simulink model "model"  (R2023a)
settings: Solver=VariableStepAuto  StartTime=0.0  StopTime=10.0  RelTol=1e-3
settings Model: Creator=Theomur  LastModifiedBy=пользователь

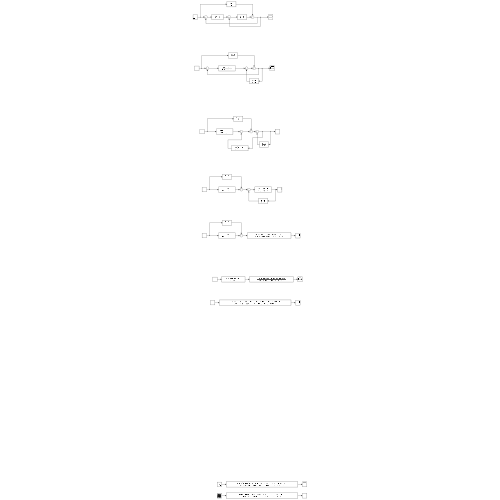
[thumbnail: Simulink's stored preview of the top-level diagram]
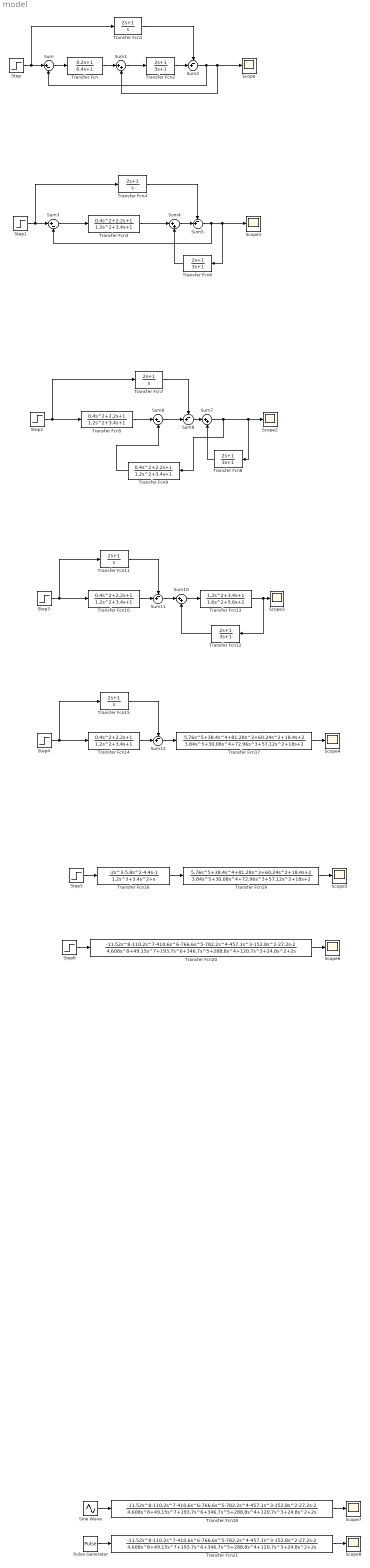
== system model ==
  Pulse Generator : DiscretePulseGenerator  PulseType=Time based  Period=10  PulseWidth=5
  Scope{,1..8} (9 alike) : Scope
  Sine Wave : Sin  SampleTime=0
  Step{,1..6} (7 alike) : Step  SampleTime=0
  Sum : Sum  Inputs=|+-
  Sum{1,4,7,10} (4 alike) : Sum  Inputs=|++
  Sum{2,5,8,11..12} (5 alike) : Sum  Inputs=-+|
  Sum3 : Sum  Inputs=|+-
  Sum6 : Sum  Inputs=|+-
  Transfer Fcn : TransferFcn  Numerator=[0.2 1]  Denominator=[0.4 1]
  Transfer Fcn{1,4,7,11,15} (5 alike) : TransferFcn  Numerator=[2 1]  Denominator=[1 0]
  Transfer Fcn{3,5,9..10,14} (5 alike) : TransferFcn  Numerator=[0.4 2.2 1]  Denominator=[1.2 3.4 1]
  Transfer Fcn{2,6,8,12} (4 alike) : TransferFcn  Numerator=[2 1]  Denominator=[3 1]
  Transfer Fcn13 : TransferFcn  Numerator=[1.2 3.4 1]  Denominator=[1.6 5.6 2]
  Transfer Fcn16 : TransferFcn  Numerator=[-2 -5.8 -4.4 -1]  Denominator=[1.2 3.4 1 0]
  Transfer Fcn17 : TransferFcn  Numerator=[5.76 38.4 81.28 60.24 18.4 2]  Denominator=[3.84 30.08 72.96 57.12 18 2]
  Transfer Fcn18 : TransferFcn  Numerator=[-11.52 -110.2 -410.6 -766.6 -782.2 -457.1 -152.8 -27.2 -2]  Denominator=[4.608 49.15 193.7 346.7 288.8 120.7 24.8 2 0]
  Transfer Fcn19 : TransferFcn  Numerator=[5.76 38.4 81.28 60.24 18.4 2]  Denominator=[3.84 30.08 72.96 57.12 18 2]
  Transfer Fcn20 : TransferFcn  Numerator=[-11.52 -110.2 -410.6 -766.6 -782.2 -457.1 -152.8 -27.2 -2]  Denominator=[4.608 49.15 193.7 346.7 288.8 120.7 24.8 2 0]
  Transfer Fcn21 : TransferFcn  Numerator=[-11.52 -110.2 -410.6 -766.6 -782.2 -457.1 -152.8 -27.2 -2]  Denominator=[4.608 49.15 193.7 346.7 288.8 120.7 24.8 2 0]
  wires:
  Step/1 -> Transfer Fcn1/1, Sum/1
  Sum/1 -> Transfer Fcn/1
  Transfer Fcn/1 -> Sum1/1
  Sum1/1 -> Transfer Fcn2/1
  Sum2/1 -> Sum/2, Scope/1, Sum1/2
  Transfer Fcn2/1 -> Sum2/2
  Transfer Fcn1/1 -> Sum2/1
  Transfer Fcn4/1 -> Sum5/1
  Sum5/1 -> Sum3/2, Transfer Fcn6/1, Scope1/1
  Step1/1 -> Transfer Fcn4/1, Sum3/1
  Sum3/1 -> Transfer Fcn3/1
  Sum4/1 -> Sum5/2
  Transfer Fcn3/1 -> Sum4/1
  Transfer Fcn6/1 -> Sum4/2
  Transfer Fcn8/1 -> Sum7/2
  Step2/1 -> Transfer Fcn7/1, Transfer Fcn5/1
  Sum7/1 -> Transfer Fcn9/1, Transfer Fcn8/1, Scope2/1
  Transfer Fcn7/1 -> Sum8/1
  Sum8/1 -> Sum7/1
  Transfer Fcn5/1 -> Sum6/1
  Sum6/1 -> Sum8/2
  Transfer Fcn9/1 -> Sum6/2
  Step3/1 -> Transfer Fcn11/1, Transfer Fcn10/1
  Transfer Fcn12/1 -> Sum10/2
  Transfer Fcn11/1 -> Sum11/1
  Sum10/1 -> Transfer Fcn13/1
  Transfer Fcn10/1 -> Sum11/2
  Sum11/1 -> Sum10/1
  Transfer Fcn13/1 -> Transfer Fcn12/1, Scope3/1
  Sum12/1 -> Transfer Fcn17/1
  Transfer Fcn14/1 -> Sum12/2
  Transfer Fcn15/1 -> Sum12/1
  Transfer Fcn17/1 -> Scope4/1
  Step4/1 -> Transfer Fcn15/1, Transfer Fcn14/1
  Step5/1 -> Transfer Fcn16/1
  Transfer Fcn19/1 -> Scope5/1
  Transfer Fcn16/1 -> Transfer Fcn19/1
  Step6/1 -> Transfer Fcn20/1
  Transfer Fcn20/1 -> Scope6/1
  Sine Wave/1 -> Transfer Fcn18/1
  Transfer Fcn18/1 -> Scope7/1
  Transfer Fcn21/1 -> Scope8/1
  Pulse Generator/1 -> Transfer Fcn21/1
